simulink model "FOC"  (R2024b)
settings: Solver=FixedStepAuto  StartTime=0.0  StopTime=2.4  FixedStep=1e-5  RelTol=1e-3
values from neighbouring files (symbols this model uses):
  dam = 0.707    [data_foc_fpc_zhang.mat]
  gama = 0.9    [data_foc_fpc_zhang.mat]
  imd = [-200 -190 -180 -170 -160 -150 -140 -130 -120 -110 -100 -90 ... (41 elements, 1x41)]    [data_foc_fpc_zhang.mat]
  imq = [-200 -180 -160 -140 -120 -100 -80 -60 -40 -20 0 20 ... (21 elements, 1x21)]    [data_foc_fpc_zhang.mat]
  L_loss = 0.0001    [data_foc_fpc_zhang.mat]
  Lmidd = [0.0012418475022 0.00124844926594 0.00125505102968 0.00126370970426 0.00127249900958 0.00128126693334 0.00129343475618 0.00129881592306 0.00130559003385 0.00130625690774 0.00129596814237 0.00127902455887 ... (861 elements, 41x21)]    [data_foc_fpc_zhang.mat]
  Lmidq = [-8.03588800241e-05 -7.81376313538e-05 -7.59163826835e-05 -6.79567507785e-05 -6.10868587727e-05 -5.46820183962e-05 -4.43623922788e-05 -2.78718084301e-05 -1.24477686412e-05 4.13620151953e-06 2.37103656882e-05 4.4707150748e-05 ... (861 elements, 41x21)]    [data_foc_fpc_zhang.mat]
  Lmiqq = [0.000622544120709 0.000618884908772 0.000615225696834 0.000593520125188 0.000579858645255 0.000568946837315 0.000562248369566 0.000560456845994 0.000560437513873 0.000561933244764 0.00056023385138 0.000557379247045 ... (861 elements, 41x21)]    [data_foc_fpc_zhang.mat]
  phase_number = 3    [data_foc_fpc_zhang.mat]
  pp = 4    [data_foc_fpc_zhang.mat]
  Psid = [-0.0498528002107 -0.0378839484092 -0.0259882808465 -0.013034575748 3.54716858652e-05 0.0129865277943 0.0255980427761 0.0386444323153 0.0516254468728 0.0646548336102 0.0777195684651 0.0905974700702 ... (861 elements, 41x21)]    [data_foc_fpc_zhang.mat]
  Psiq = [-0.428836914229 -0.429385909203 -0.42997932915 -0.43118839194 -0.431809140992 -0.432336580454 -0.433057103512 -0.432963079787 -0.433296951787 -0.433632934983 -0.43343561964 -0.433301309559 ... (861 elements, 41x21)]    [data_foc_fpc_zhang.mat]
  Rs = 0.015    [data_foc_fpc_zhang.mat]
  T_ref = 162    [data_foc_fpc_zhang.mat]
  Ts = 1e-05    [data_foc_fpc_zhang.mat]
undefined symbols (not defined in the file or in its folder): DiscIntNeverNeededParam, UNC, V_dc
libraries: simulink x7, spsabctodq0Lib x2, spsdq0toabcLib x2, simulink_extras x2, mcbcontrolslib x2, mcbplantlib x1
settings Model: Creator=zhang5  LastModifiedBy=zhang5
settings DataIOCC: ReturnWorkspaceOutputs=off

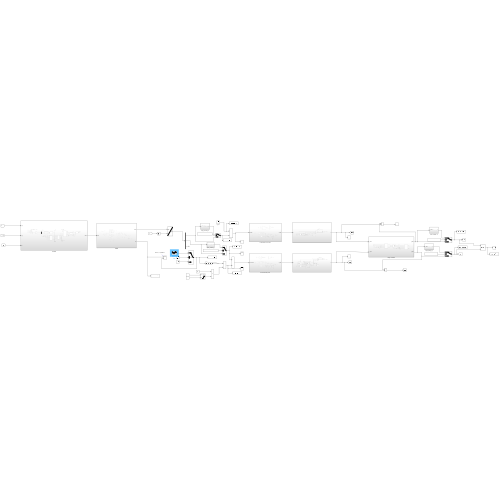
[thumbnail: Simulink's stored preview of the top-level diagram]
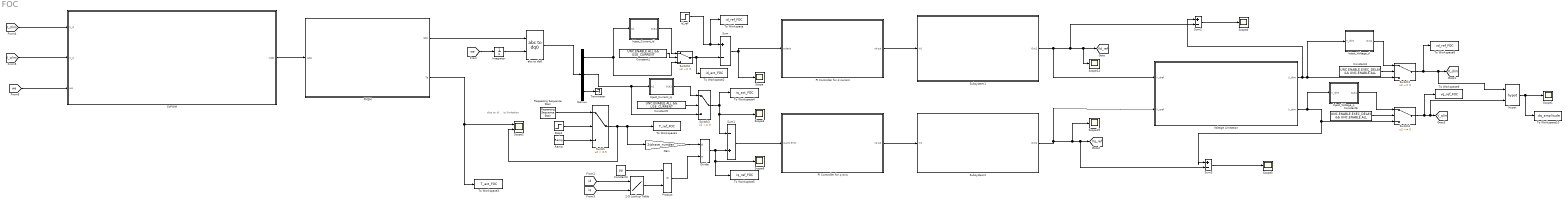
== system FOC ==
  note: due to id ， iq limitation
  2-D Lookup Table : Lookup_n-D  BreakpointsForDimension1=imd  BreakpointsForDimension2=imq  Table=Psid  InternalRulePriority=Speed  RndMeth=Simplest
      settings: InputPortMap=u0,u1
  Constant1 : Constant  Value="UNC.ENABLE.ALL   && USE_CURRENT"
  Constant3 : Constant  Value=pp
  Constant4 : Constant  Value="UNC.ENABLE.EXEC_DELAY &&  UNC.ENABLE.ALL"
  Constant5 : Constant  Value="UNC.ENABLE.ALL   && USE_CURRENT"
  Constant6 : Constant  Value=UNC.ENABLE.EXEC_DELAY && UNC.ENABLE.ALL
  Demux : Demux  Outputs=3
  Divide : Product  Inputs=*/
  Gain : Gain  Gain=2/phase_number
  Hypot : Math  Operator=hypot
  Inject_Current_id : Subsystem
  Inject_Current_iq : Subsystem
  Inject_Voltage_d : Subsystem
  Inject_Voltage_q : Subsystem
  Integrator : Integrator
  "PI Controller for d current " : Subsystem
  "PI Controller for q axis " : Subsystem
  PMSM : Subsystem
  Product : Product
  Ramp : simulink/Sources/Ramp  slope=90  start=0  InitialOutput=0
  Repeating Sequence Stair : simulink/Sources/Repeating Sequence Stair  OutValues="[T_ref  -T_ref*0.3 -T_ref*1.8 -T_ref T_ref*1.8 T_ref*0.1].'"  tsamp=0.4  OutMin=[]  OutMax=[]  OutDataTypeStr=double  OutputDataTypeScalingMode=double  OutDataType=fixdt(0,8)  ConRadixGroup=Best Precision: Vector-wise  OutScaling=2^-12
  SVPWM : Subsystem
  Scope{,1,3..6,14..15} (8 alike) : Scope
  Scope2 : Scope  NumInputPorts=2
  Step1 : Step  Time=5  SampleTime=0
  Subsystem1 : Subsystem
  Subsystem2 : Subsystem
  Sum : Sum  Inputs=+-
  Sum1 : Sum  Inputs=-+
  Sum2 : Sum  Inputs=+-
  Sum3 : Sum  Inputs=+-
  Switch : Switch  Criteria=u2 > Threshold  Threshold=0.5  SaturateOnIntegerOverflow=off  InputSameDT=off
  Switch{1..4} (4 alike) : Switch  Criteria=u2 ~= 0  SaturateOnIntegerOverflow=off  InputSameDT=off
  Terminator : Terminator
  To Workspace : ToWorkspace  VariableName=id_ref_FOC  SaveFormat=Structure With Time  SampleTime=-1
  To Workspace1 : ToWorkspace  VariableName=T_ref_FOC  SaveFormat=Structure With Time  SampleTime=-1
  To Workspace10 : ToWorkspace  VariableName=dq_amplitude  SaveFormat=Structure With Time  SampleTime=-1
  To Workspace2 : ToWorkspace  VariableName=id_act_FOC  SaveFormat=Structure With Time  SampleTime=-1
  To Workspace3 : ToWorkspace  VariableName=T_act_FOC  SaveFormat=Structure With Time  SampleTime=-1
  To Workspace4 : ToWorkspace  VariableName=iq_act_FOC  SaveFormat=Structure With Time  SampleTime=-1
  To Workspace5 : ToWorkspace  VariableName=iq_ref_FOC  SaveFormat=Structure With Time  SampleTime=-1
  To Workspace8 : ToWorkspace  VariableName=vd_ref_FOC  SaveFormat=Structure With Time  SampleTime=-1
  To Workspace9 : ToWorkspace  VariableName=vq_ref_FOC  SaveFormat=Structure With Time  SampleTime=-1
  Voltage Limitation : Subsystem
  abc to dq0 : spsabctodq0Lib/abc to dq0  Alignment=Aligned with phase A axis
  id_ref : Step  Time=4  After=0  SampleTime=0
  tag scope: V_dlim=global, V_qlim=global, Vd_ref=global, Vq_ref=global
  wires:
  [we] -> Integrator/1
  Integrator/1 -> abc to dq0/2
  abc to dq0/1 -> Demux/1
  Demux/3 -> Terminator/1
  Gain/1 -> Divide/1
  Constant3/1 -> Product/1
  [id] -> 2-D Lookup Table/1
  [iq] -> 2-D Lookup Table/2
  Product/1 -> Divide/2
  Sum/1 -> Scope/1, "PI Controller for d current "/1(e daxis)
  Sum1/1 -> "PI Controller for q axis "/1(q axis error)
  "PI Controller for d current "/1(vd out) -> Subsystem1/1(In1)
  Subsystem1/1(Out1) -> Sum2/2, Scope14/1, [Vd_ref], Voltage Limitation/1(V_dref)
  "PI Controller for q axis "/1(vq out) -> Subsystem2/1(In1)
  Voltage Limitation/1(V_dlim) -> Sum2/1, Inject_Voltage_d/1(V_dlim), Switch1/3
  Sum2/1 -> Scope4/1
  Sum3/1 -> Scope5/1
  Voltage Limitation/2(V_qlim) -> Inject_Voltage_q/1(V_dlim), Switch4/3, Sum3/1
  Subsystem2/1(Out1) -> Voltage Limitation/2(V_qref), Scope15/1, Sum3/2, [Vq_ref]
  Step1/1 -> Switch/2
  PMSM/2(Te) -> Scope2/1, To Workspace3/1
  id_ref/1 -> To Workspace/1, Sum/1
  Ramp/1 -> Switch/3
  Switch/1 -> Gain/1, To Workspace1/1, Scope2/2
  PMSM/1(iabc) -> abc to dq0/1
  Constant4/1 -> Switch1/2
  Demux/1 -> Inject_Current_id/1(In1), Switch2/3
  Demux/2 -> Switch3/3, Inject_Current_iq/1(In1)
  Constant1/1 -> Switch2/2
  Inject_Current_id/1(Out1) -> Switch2/1
  Inject_Current_iq/1(Out1) -> Switch3/1
  Constant5/1 -> Switch3/2
  Inject_Voltage_d/1(Out1) -> Switch1/1
  Inject_Voltage_q/1(Out1) -> Switch4/1
  Constant6/1 -> Switch4/2
  Switch2/1 -> To Workspace2/1, Sum/2
  Switch3/1 -> To Workspace4/1, Scope3/1, Sum1/1
  Switch1/1 -> To Workspace8/1, Hypot/1, [V_dlim]
  Switch4/1 -> To Workspace9/1, Hypot/2, [V_qlim]
  Divide/1 -> Scope6/1, To Workspace5/1, Sum1/2
  Repeating Sequence Stair/1 -> Switch/1
  [V_dlim] -> SVPWM/1(V_d)
  [V_qlim] -> SVPWM/2(V_q)
  [we] -> SVPWM/3(we)
  SVPWM/1(Vabc) -> PMSM/1(vabc)
  Hypot/1 -> To Workspace10/1, Scope1/1
  2-D Lookup Table/1 -> Product/2

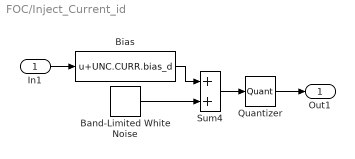
== system FOC/Inject_Current_id ==
  In1 : Inport
  Band-Limited White Noise : simulink/Sources/Band-Limited White Noise  Cov=UNC.CURR.noise_psd  Ts=1e-5  seed=[23341]
  Bias : Bias  Bias=UNC.CURR.bias_d  SaturateOnIntegerOverflow=off
  Quantizer : Quantizer  QuantizationInterval=UNC.CURR.quant
  Sum4 : Sum
  Out1 : Outport
  wires:
  Sum4/1 -> Quantizer/1
  Quantizer/1 -> Out1/1
  In1/1 -> Bias/1
  Bias/1 -> Sum4/1
  Band-Limited White Noise/1 -> Sum4/2

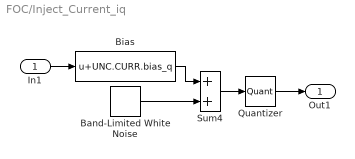
== system FOC/Inject_Current_iq ==
  In1 : Inport
  Band-Limited White Noise : simulink/Sources/Band-Limited White Noise  Cov=UNC.CURR.noise_psd  Ts=1e-5  seed=[23341]
  Bias : Bias  Bias=UNC.CURR.bias_q  SaturateOnIntegerOverflow=off
  Quantizer : Quantizer  QuantizationInterval=UNC.CURR.quant
  Sum4 : Sum
  Out1 : Outport
  wires:
  Band-Limited White Noise/1 -> Sum4/2
  Bias/1 -> Sum4/1
  In1/1 -> Bias/1
  Quantizer/1 -> Out1/1
  Sum4/1 -> Quantizer/1

== system FOC/Inject_Voltage_d ==
  V_dlim : Inport
  Transport Delay : TransportDelay  DelayTime=UNC.DELAY.ctrl
  Out1 : Outport
  wires:
  V_dlim/1 -> Transport Delay/1
  Transport Delay/1 -> Out1/1

== system FOC/Inject_Voltage_q ==
  V_dlim : Inport
  Transport Delay : TransportDelay  DelayTime=UNC.DELAY.ctrl
  Out1 : Outport
  wires:
  Transport Delay/1 -> Out1/1
  V_dlim/1 -> Transport Delay/1

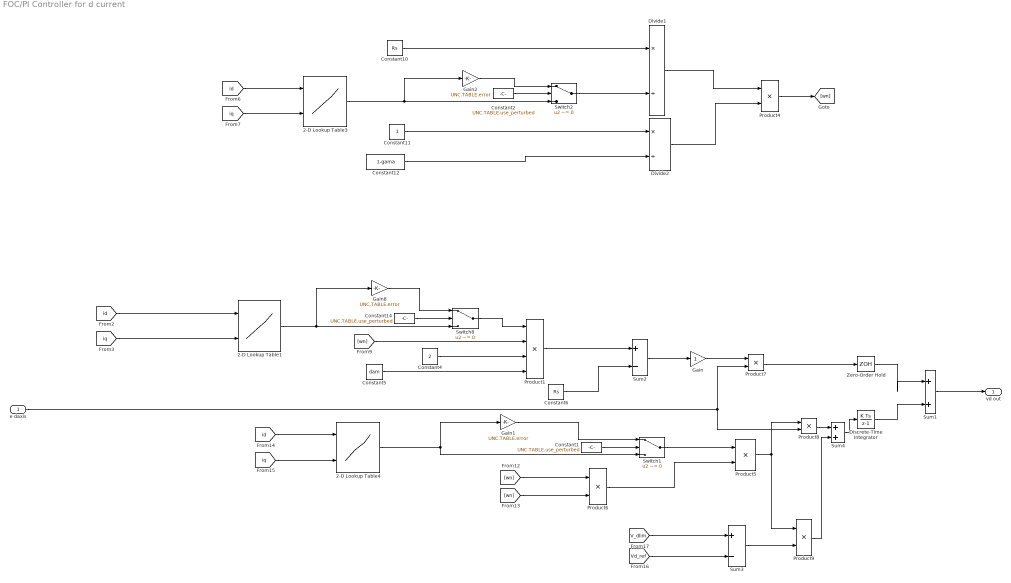
== system FOC/PI Controller for d current  ==
  e daxis : Inport
  2-D Lookup Table1 : Lookup_n-D  BreakpointsForDimension1=imd  BreakpointsForDimension2=imq  Table=Lmidd  InternalRulePriority=Speed  RndMeth=Simplest
      settings: InputPortMap=u0,u1
  2-D Lookup Table3 : Lookup_n-D  BreakpointsForDimension1=imd  BreakpointsForDimension2=imq  Table=Lmidd  InternalRulePriority=Speed  RndMeth=Simplest
      settings: InputPortMap=u0,u1
  2-D Lookup Table4 : Lookup_n-D  BreakpointsForDimension1=imd  BreakpointsForDimension2=imq  Table=Lmidd  InternalRulePriority=Speed  RndMeth=Simplest
      settings: InputPortMap=u0,u1
  Constant1 : Constant  Value=UNC.TABLE.use_perturbed
  Constant10 : Constant  Value=Rs
  Constant11 : Constant
  Constant12 : Constant  Value=1-gama
  Constant14 : Constant  Value=UNC.TABLE.use_perturbed
  Constant2 : Constant  Value=UNC.TABLE.use_perturbed
  Constant4 : Constant  Value=2
  Constant5 : Constant  Value=dam
  Constant6 : Constant  Value=Rs
  Discrete-Time Integrator : DiscreteIntegrator  SampleTime=Ts  ICPrevOutput=DiscIntNeverNeededParam  ICPrevScaledInput=DiscIntNeverNeededParam
  Divide1 : Product  Inputs=*/
  Divide2 : Product  Inputs=*/
  Gain : Gain
  Gain1 : Gain  Gain=UNC.TABLE.error
  Gain2 : Gain  Gain=UNC.TABLE.error
  Gain8 : Gain  Gain=UNC.TABLE.error
  Product1 : Product  Inputs=4
  Product{4..9} (6 alike) : Product
  Sum1 : Sum  Inputs=|++
  Sum2 : Sum  Inputs=+-
  Sum3 : Sum  Inputs=+-
  Sum4 : Sum
  Switch1 : Switch  Criteria=u2 ~= 0  SaturateOnIntegerOverflow=off  InputSameDT=off
  Switch2 : Switch  Criteria=u2 ~= 0  SaturateOnIntegerOverflow=off  InputSameDT=off
  Switch8 : Switch  Criteria=u2 ~= 0  SaturateOnIntegerOverflow=off  InputSameDT=off
  Zero-Order Hold : ZeroOrderHold  SampleTime=Ts
  vd out : Outport
  wires:
  Constant12/1 -> Divide2/2
  Divide2/1 -> Product4/2
  Constant11/1 -> Divide2/1
  Product4/1 -> [wn]
  Divide1/1 -> Product4/1
  [id] -> 2-D Lookup Table3/1
  [iq] -> 2-D Lookup Table3/2
  Constant10/1 -> Divide1/1
  Zero-Order Hold/1 -> Sum1/1
  Discrete-Time Integrator/1 -> Sum1/2
  Product1/1 -> Sum2/1
  Constant4/1 -> Product1/3
  Constant5/1 -> Product1/4
  [wn] -> Product1/2
  [id] -> 2-D Lookup Table1/1
  Constant6/1 -> Sum2/2
  [iq] -> 2-D Lookup Table1/2
  [id] -> 2-D Lookup Table4/1
  [wn] -> Product6/2
  Product6/1 -> Product5/2
  [iq] -> 2-D Lookup Table4/2
  [wn] -> Product6/1
  Sum2/1 -> Gain/1
  Product7/1 -> Zero-Order Hold/1
  Product5/1 -> Product9/1, Product8/1
  e daxis/1 -> Product7/2, Product8/2
  Sum1/1 -> vd out/1
  [Vd_ref] -> Sum3/2
  [V_dlim] -> Sum3/1
  Sum3/1 -> Product9/2
  Product8/1 -> Sum4/1
  Product9/1 -> Sum4/2
  Sum4/1 -> Discrete-Time Integrator/1
  Gain/1 -> Product7/1
  Constant14/1 -> Switch8/2
  Gain8/1 -> Switch8/1
  2-D Lookup Table1/1 -> Gain8/1, Switch8/3
  Switch8/1 -> Product1/1
  Switch1/1 -> Product5/1
  2-D Lookup Table4/1 -> Switch1/3, Gain1/1
  Gain1/1 -> Switch1/1
  Constant1/1 -> Switch1/2
  Switch2/1 -> Divide1/2
  2-D Lookup Table3/1 -> Switch2/3, Gain2/1
  Gain2/1 -> Switch2/1
  Constant2/1 -> Switch2/2

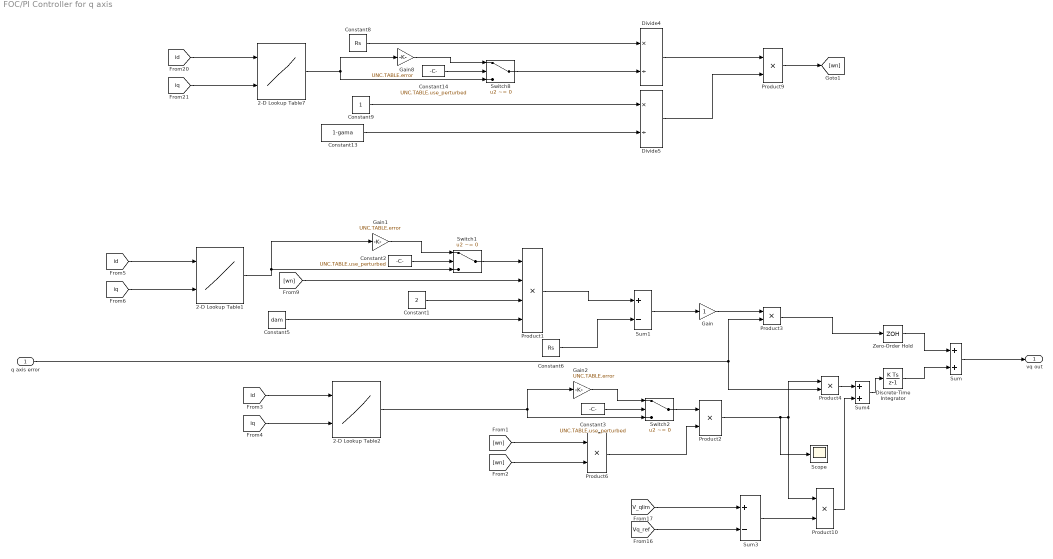
== system FOC/PI Controller for q axis  ==
  q axis error : Inport
  2-D Lookup Table1 : Lookup_n-D  BreakpointsForDimension1=imd  BreakpointsForDimension2=imq  Table=Lmiqq  InternalRulePriority=Speed  RndMeth=Simplest
      settings: InputPortMap=u0,u1
  2-D Lookup Table2 : Lookup_n-D  BreakpointsForDimension1=imd  BreakpointsForDimension2=imq  Table=Lmiqq  InternalRulePriority=Speed  RndMeth=Simplest
      settings: InputPortMap=u0,u1
  2-D Lookup Table7 : Lookup_n-D  BreakpointsForDimension1=imd  BreakpointsForDimension2=imq  Table=Lmiqq  InternalRulePriority=Speed  RndMeth=Simplest
      settings: InputPortMap=u0,u1
  Constant1 : Constant  Value=2
  Constant13 : Constant  Value=1-gama
  Constant14 : Constant  Value=UNC.TABLE.use_perturbed
  Constant2 : Constant  Value=UNC.TABLE.use_perturbed
  Constant3 : Constant  Value=UNC.TABLE.use_perturbed
  Constant5 : Constant  Value=dam
  Constant6 : Constant  Value=Rs
  Constant8 : Constant  Value=Rs
  Constant9 : Constant
  Discrete-Time Integrator : DiscreteIntegrator  SampleTime=Ts  ICPrevOutput=DiscIntNeverNeededParam  ICPrevScaledInput=DiscIntNeverNeededParam
  Divide4 : Product  Inputs=*/
  Divide5 : Product  Inputs=*/
  Gain : Gain
  Gain1 : Gain  Gain=UNC.TABLE.error
  Gain2 : Gain  Gain=UNC.TABLE.error
  Gain8 : Gain  Gain=UNC.TABLE.error
  Product1 : Product  Inputs=4
  Product{2..4,6,9..10} (6 alike) : Product
  Scope : Scope
  Sum : Sum
  Sum1 : Sum  Inputs=+-
  Sum3 : Sum  Inputs=+-
  Sum4 : Sum
  Switch1 : Switch  Criteria=u2 ~= 0  SaturateOnIntegerOverflow=off  InputSameDT=off
  Switch2 : Switch  Criteria=u2 ~= 0  SaturateOnIntegerOverflow=off  InputSameDT=off
  Switch8 : Switch  Criteria=u2 ~= 0  SaturateOnIntegerOverflow=off  InputSameDT=off
  Zero-Order Hold : ZeroOrderHold  SampleTime=Ts
  vq out : Outport
  wires:
  Constant13/1 -> Divide5/2
  Divide4/1 -> Product9/1
  Product9/1 -> [wn]
  Constant9/1 -> Divide5/1
  [id] -> 2-D Lookup Table7/1
  Constant8/1 -> Divide4/1
  Divide5/1 -> Product9/2
  [iq] -> 2-D Lookup Table7/2
  Sum4/1 -> Discrete-Time Integrator/1
  q axis error/1 -> Product4/2, Product3/2
  Zero-Order Hold/1 -> Sum/1
  Constant6/1 -> Sum1/2
  Discrete-Time Integrator/1 -> Sum/2
  Constant5/1 -> Product1/4
  Constant1/1 -> Product1/3
  [wn] -> Product1/2
  Product1/1 -> Sum1/1
  Sum3/1 -> Product10/2
  Product2/1 -> Scope/1, Product10/1, Product4/1
  [V_qlim] -> Sum3/1
  Product10/1 -> Sum4/2
  Sum1/1 -> Gain/1
  [Vq_ref] -> Sum3/2
  [wn] -> Product6/2
  [wn] -> Product6/1
  Product6/1 -> Product2/2
  Product4/1 -> Sum4/1
  Product3/1 -> Zero-Order Hold/1
  [iq] -> 2-D Lookup Table1/2
  [id] -> 2-D Lookup Table1/1
  [iq] -> 2-D Lookup Table2/2
  [id] -> 2-D Lookup Table2/1
  Sum/1 -> vq out/1
  Gain/1 -> Product3/1
  Constant14/1 -> Switch8/2
  Gain8/1 -> Switch8/1
  2-D Lookup Table7/1 -> Gain8/1, Switch8/3
  Switch8/1 -> Divide4/2
  2-D Lookup Table1/1 -> Gain1/1, Switch1/3
  Gain1/1 -> Switch1/1
  Constant2/1 -> Switch1/2
  Constant3/1 -> Switch2/2
  Gain2/1 -> Switch2/1
  2-D Lookup Table2/1 -> Switch2/3, Gain2/1
  Switch2/1 -> Product2/1
  Switch1/1 -> Product1/1

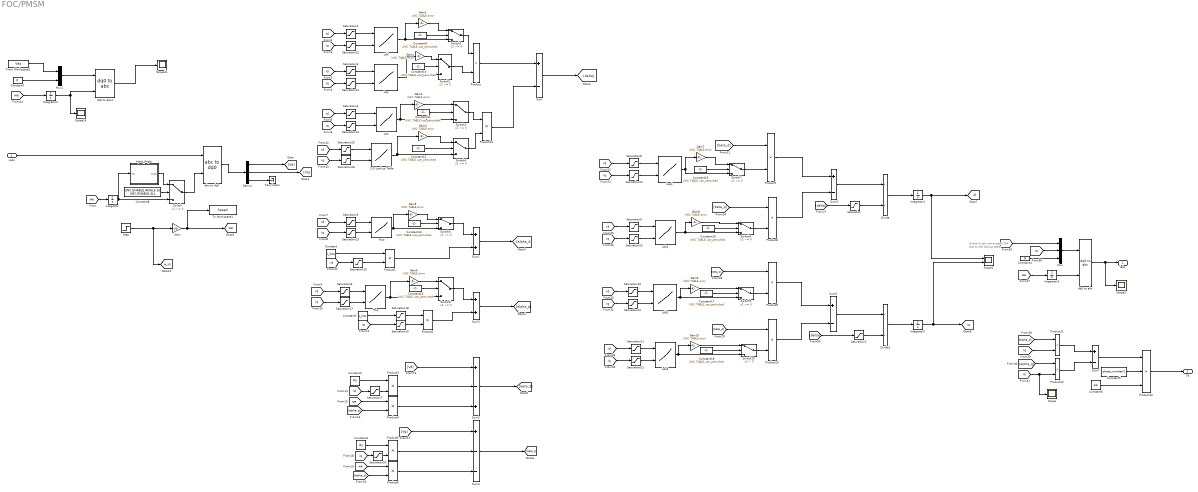
== system FOC/PMSM ==
  note: id and iq can not exceed 200
      | due to the lookup table
  vabc : Inport
  2-D Lookup Table : Lookup_n-D  BreakpointsForDimension1=imd  BreakpointsForDimension2=imq  Table=Lmidq  ExtrapMethod=Clip  UseLastTableValue=on  InternalRulePriority=Speed  RndMeth=Simplest
      settings: InputPortMap=u0,u1
  Constant : Constant  Value=L_loss
  Constant1 : Constant  Value=L_loss
  Constant{9..18} (10 alike) : Constant  Value=UNC.TABLE.use_perturbed
  Constant2 : Constant  Value=Rs
  Constant3 : Constant  Value=Rs
  Constant4 : Constant  Value=0
  Constant5 : Constant  Value=phase_number/2
  Constant6 : Constant  Value=pp
  Constant7 : Constant  Value=0
  Constant8 : Constant  Value=UNC.ENABLE.ANGLE && UNC.ENABLE.ALL
  Demux : Demux  Outputs=3
  Divide : Product  Inputs=*/
  Divide1 : Product  Inputs=*/
  From Workspace2 : FromWorkspace  VariableName=Vdq  SampleTime=1e-5  Interpolate=off  OutputAfterFinalValue=Holding final value
  Gain : Gain  Gain=pp
  Gain{1..10} (10 alike) : Gain  Gain=UNC.TABLE.error
  Inject_Angle : Subsystem
  Integrator : Integrator  UpperSaturationLimit=pi  LowerSaturationLimit=-pi
  Integrator1 : Integrator
  Integrator2 : Integrator
  Integrator3 : Integrator  UpperSaturationLimit=pi  LowerSaturationLimit=-pi
  Integrator4 : Integrator  UpperSaturationLimit=pi  LowerSaturationLimit=-pi
  Ldd : Lookup_n-D  BreakpointsForDimension1=imd  BreakpointsForDimension2=imq  Table=Lmidd  ExtrapMethod=Clip  UseLastTableValue=on  InternalRulePriority=Speed  RndMeth=Simplest
      settings: InputPortMap=u0,u1
  Ldd1 : Lookup_n-D  BreakpointsForDimension1=imd  BreakpointsForDimension2=imq  Table=Lmidd  ExtrapMethod=Clip  UseLastTableValue=on  InternalRulePriority=Speed  RndMeth=Simplest
      settings: InputPortMap=u0,u1
  Ldq : Lookup_n-D  BreakpointsForDimension1=imd  BreakpointsForDimension2=imq  Table=Lmidq  ExtrapMethod=Clip  UseLastTableValue=on  InternalRulePriority=Speed  RndMeth=Simplest
      settings: InputPortMap=u0,u1
  Ldq1 : Lookup_n-D  BreakpointsForDimension1=imd  BreakpointsForDimension2=imq  Table=Lmidq  ExtrapMethod=Clip  UseLastTableValue=on  InternalRulePriority=Speed  RndMeth=Simplest
      settings: InputPortMap=u0,u1
  Ldq2 : Lookup_n-D  BreakpointsForDimension1=imd  BreakpointsForDimension2=imq  Table=Lmidq  ExtrapMethod=Clip  UseLastTableValue=on  InternalRulePriority=Speed  RndMeth=Simplest
      settings: InputPortMap=u0,u1
  Lqq : Lookup_n-D  BreakpointsForDimension1=imd  BreakpointsForDimension2=imq  Table=Lmiqq  ExtrapMethod=Clip  UseLastTableValue=on  InternalRulePriority=Speed  RndMeth=Simplest
      settings: InputPortMap=u0,u1
  Lqq1 : Lookup_n-D  BreakpointsForDimension1=imd  BreakpointsForDimension2=imq  Table=Lmiqq  ExtrapMethod=Clip  UseLastTableValue=on  InternalRulePriority=Speed  RndMeth=Simplest
      settings: InputPortMap=u0,u1
  Mux : Mux  Inputs=3
  Mux1 : Mux  Inputs=2
  Product{,1..12,14} (14 alike) : Product
  Product13 : Product  Inputs=3
  Psid : Lookup_n-D  BreakpointsForDimension1=imd  BreakpointsForDimension2=imq  Table=Psid  ExtrapMethod=Clip  UseLastTableValue=on  InternalRulePriority=Speed  RndMeth=Simplest
      settings: InputPortMap=u0,u1
  Psiq : Lookup_n-D  BreakpointsForDimension1=imd  BreakpointsForDimension2=imq  Table=Psiq  ExtrapMethod=Clip  UseLastTableValue=on  InternalRulePriority=Speed  RndMeth=Simplest
      settings: InputPortMap=u0,u1
  Saturation : Saturate  UpperLimit=10000000000000000000000  LowerLimit=1e-6
  Saturation1 : Saturate  UpperLimit=10000000000000000000000  LowerLimit=1e-6
  Saturation{2..11,13..26} (24 alike) : Saturate  UpperLimit=200  LowerLimit=-200
  Saturation12 : Saturate
  Scope{,2,11,14} (4 alike) : Scope
  Scope1 : Scope  NumInputPorts=2
  Step : Step  Time=5  Before=10.4720  After=10.4720*1.2  SampleTime=0
  Sum{,5..7} (4 alike) : Sum  Inputs=+-
  Sum1 : Sum
  Sum2 : Sum
  Sum3 : Sum  Inputs=+-+
  Sum4 : Sum  Inputs=+--
  Switch{,1..9} (10 alike) : Switch  Criteria=u2 ~= 0  SaturateOnIntegerOverflow=off  InputSameDT=off
  Switch10 : Switch  Criteria=u2 > Threshold  SaturateOnIntegerOverflow=off  InputSameDT=off
  Terminator : Terminator
  To Workspace1 : ToWorkspace  VariableName=Speed  SaveFormat=Structure With Time  SampleTime=-1
  abc to dq0 : spsabctodq0Lib/abc to dq0  Alignment=Aligned with phase A axis
  dq0 to abc : spsdq0toabcLib/dq0 to abc  Alignment=Aligned with phase A axis
  dq0 to abc1 : spsdq0toabcLib/dq0 to abc  Alignment=Aligned with phase A axis
  iabc : Outport
  Te : Outport  Port=2
  tag scope: id=global, iq=global, w_m=global, we=global
  wires:
  [iq] -> Saturation17/1
  [iq] -> Saturation12/1
  [iq] -> Saturation21/1
  Constant2/1 -> Product3/1
  Product4/1 -> Sum3/3
  [iq] -> Saturation19/1
  [iq] -> Saturation15/1
  [id] -> Saturation16/1
  Constant3/1 -> Product5/1
  [id] -> Saturation2/1
  [beta_d] -> Product10/1
  [we] -> Integrator/1
  [id] -> Saturation10/1
  Demux/3 -> Terminator/1
  dq0 to abc/1 -> Scope2/1, iabc/1
  Constant4/1 -> Mux/3
  [id] -> Saturation6/1
  [Vq] -> Sum4/1
  Divide1/1 -> Integrator2/1
  [alpha_d] -> Product6/2
  [iq] -> Saturation14/1
  Mux/1 -> dq0 to abc/1
  [id] -> Saturation9/1
  Product6/1 -> Sum4/3
  [iq] -> Saturation13/1
  [id] -> Saturation3/1
  [iq] -> Saturation24/1
  Product7/1 -> Sum5/1
  Sum2/1 -> [alpha_q]
  Product14/1 -> Sum/2
  [id] -> Saturation4/1
  [iq] -> Saturation20/1
  [we] -> Integrator3/1
  [delta] -> Saturation/1
  [id] -> Saturation7/1
  Sum5/1 -> Divide/1
  Product8/1 -> Sum5/2
  Product3/1 -> Sum3/2
  Gain/1 -> To Workspace1/1, [we]
  [beta_q] -> Product8/1
  Integrator3/1 -> dq0 to abc/2
  [beta_d] -> Product7/1
  [id] -> Saturation8/1
  [iq] -> Mux/2
  Divide/1 -> Integrator1/1
  Product9/1 -> Sum6/1
  Product5/1 -> Sum4/2
  Constant1/1 -> Saturation18/1
  Product10/1 -> Sum6/2
  [id] -> Mux/1
  [we] -> Product4/1
  [iq] -> Saturation23/1
  Product/1 -> Sum/1
  Sum6/1 -> Divide1/1
  [we] -> Product6/1
  Sum3/1 -> [beta_d]
  [alpha_q] -> Product4/2
  Sum4/1 -> [beta_q]
  Sum1/1 -> [alpha_d]
  [id] -> Saturation11/1
  [id] -> Saturation5/1
  [Vd] -> Sum3/1
  [delta] -> Saturation1/1
  Integrator1/1 -> Scope1/1, [id]
  Constant/1 -> Product1/1
  Sum/1 -> [delta]
  [iq] -> Saturation22/1
  [beta_q] -> Product9/1
  [alpha_d] -> Product11/1
  [iq] -> Product11/2
  Product11/1 -> Sum7/1
  [alpha_q] -> Product12/1
  [id] -> Scope/1, Product12/2
  Product12/1 -> Sum7/2
  Sum7/1 -> Product13/1
  Constant5/1 -> Product13/2
  Constant6/1 -> Product13/3
  Product13/1 -> Te/1
  Saturation/1 -> Divide/2
  Saturation1/1 -> Divide1/2
  Saturation2/1 -> Ldd/1
  Saturation3/1 -> Lqq/1
  Saturation4/1 -> Ldq/1
  Saturation5/1 -> Psid/1
  Saturation6/1 -> Psiq/1
  Saturation7/1 -> Product3/2
  Saturation8/1 -> Lqq1/1
  Saturation9/1 -> Ldq1/1
  Saturation10/1 -> Ldd1/1
  Saturation11/1 -> Ldq2/1
  Saturation12/1 -> Ldd/2
  Saturation13/1 -> Lqq/2
  Saturation14/1 -> Ldq/2
  Saturation15/1 -> Psid/2
  Saturation16/1 -> Product1/2
  Saturation17/1 -> Psiq/2
  Saturation18/1 -> Product2/1
  Saturation19/1 -> Product2/2
  Saturation20/1 -> Product5/2
  Saturation21/1 -> Ldq2/2
  Saturation22/1 -> Ldd1/2
  Saturation23/1 -> Ldq1/2
  Saturation24/1 -> Lqq1/2
  [id] -> Saturation25/1
  [iq] -> Saturation26/1
  Saturation25/1 -> 2-D Lookup Table/1
  Saturation26/1 -> 2-D Lookup Table/2
  Product2/1 -> Sum2/2
  Demux/1 -> [Vd]
  Demux/2 -> [Vq]
  abc to dq0/1 -> Demux/1
  Product1/1 -> Sum1/2
  Mux1/1 -> dq0 to abc1/1
  Integrator4/1 -> Scope14/1, dq0 to abc1/2
  Constant7/1 -> Mux1/2
  From Workspace2/1 -> Mux1/1
  dq0 to abc1/1 -> Scope11/1
  [we] -> Integrator4/1
  vabc/1 -> abc to dq0/1
  Step/1 -> [w_m], Gain/1
  Integrator/1 -> Inject_Angle/1(In1), Switch/3
  Lqq/1 -> Gain2/1, Switch2/3
  Ldq/1 -> Gain3/1, Switch3/3
  2-D Lookup Table/1 -> Gain4/1, Switch4/3
  Psiq/1 -> Gain6/1, Switch6/3
  Lqq1/1 -> Gain7/1, Switch7/3
  Ldq1/1 -> Gain8/1, Switch8/3
  Ldd1/1 -> Gain9/1, Switch9/3
  Ldq2/1 -> Gain10/1, Switch10/3
  Inject_Angle/1(Out1) -> Switch/1
  Constant8/1 -> Switch/2
  Ldd/1 -> Gain1/1, Switch1/3
  Constant9/1 -> Switch1/2
  Gain1/1 -> Switch1/1
  Gain2/1 -> Switch2/1
  Switch2/1 -> Product/2
  Switch1/1 -> Product/1
  Constant10/1 -> Switch2/2
  Gain3/1 -> Switch3/1
  Switch3/1 -> Product14/1
  Constant11/1 -> Switch3/2
  Switch4/1 -> Product14/2
  Gain4/1 -> Switch4/1
  Constant12/1 -> Switch4/2
  Gain5/1 -> Switch5/1
  Psid/1 -> Gain5/1, Switch5/3
  Constant13/1 -> Switch5/2
  Gain6/1 -> Switch6/1
  Constant14/1 -> Switch6/2
  Switch6/1 -> Sum2/1
  Switch5/1 -> Sum1/1
  Gain7/1 -> Switch7/1
  Constant15/1 -> Switch7/2
  Gain8/1 -> Switch8/1
  Constant16/1 -> Switch8/2
  Gain9/1 -> Switch9/1
  Constant17/1 -> Switch9/2
  Switch9/1 -> Product9/2
  Switch8/1 -> Product8/2
  Switch10/1 -> Product10/2
  Gain10/1 -> Switch10/1
  Constant18/1 -> Switch10/2
  Switch7/1 -> Product7/2
  Switch/1 -> abc to dq0/2
  Integrator2/1 -> [iq], Scope1/2

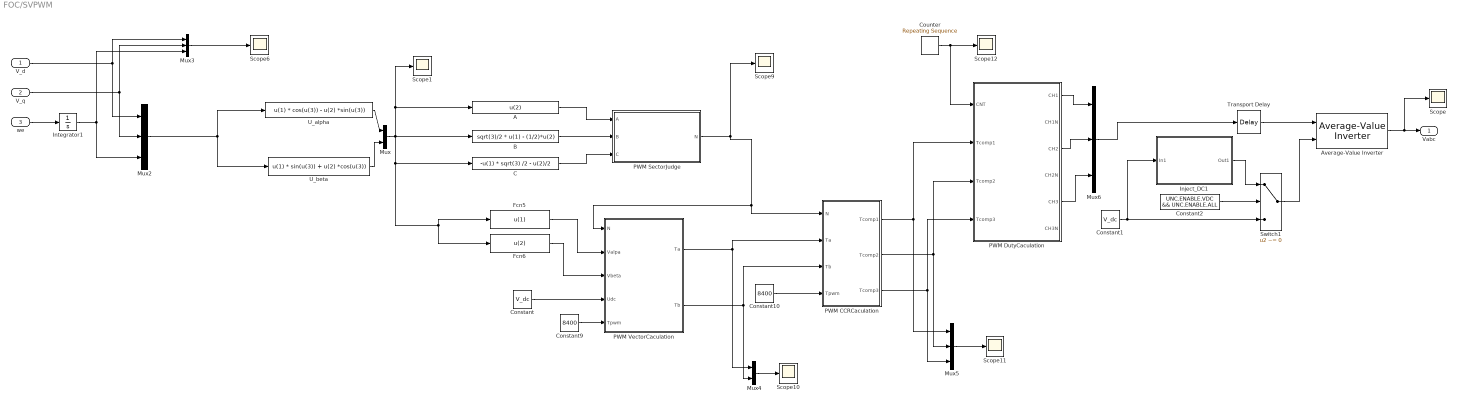
== system FOC/SVPWM ==
  V_d : Inport
  V_q : Inport  Port=2
  we : Inport  Port=3
  A : Fcn  Expr=u(2)
  Average-Value Inverter : mcbplantlib/Average-Value Inverter
      settings: LibrarySourceBlock=mcblib/Electrical Systems/Inverters/Average-Value Inverter
  B : Fcn  Expr=sqrt(3)/2 * u(1) - (1/2)*u(2)
  C : Fcn  Expr=-u(1) * sqrt(3) /2 - u(2)/2
  Constant : Constant  Value=V_dc
  Constant1 : Constant  Value=V_dc
  Constant10 : Constant  Value=8400
  Constant2 : Constant  Value=UNC.ENABLE.VDC && UNC.ENABLE.ALL
  Constant9 : Constant  Value=8400
  Counter : simulink/Sources/Repeating Sequence  rep_seq_t=[0 0.00025 0.0005]  rep_seq_y=[0 4200 0]
  Fcn5 : Fcn  Expr=u(1)
  Fcn6 : Fcn  Expr=u(2)
  Inject_DC1 : Subsystem
  Integrator1 : Integrator
  Mux : Mux  Inputs=2
  Mux{2..3,5..6} (4 alike) : Mux  Inputs=3
  Mux4 : Mux  Inputs=2
  PWM CCRCaculation : MATLAB Function  TreatAsAtomicUnit=on
  PWM DutyCaculation : MATLAB Function  TreatAsAtomicUnit=on
  PWM SectorJudge : MATLAB Function  TreatAsAtomicUnit=on
  PWM VectorCaculation : MATLAB Function  TreatAsAtomicUnit=on
  Scope{,1,6,9..12} (7 alike) : Scope
  Switch1 : Switch  Criteria=u2 ~= 0  SaturateOnIntegerOverflow=off  InputSameDT=off
  Transport Delay : TransportDelay  DelayTime=UNC.DELAY.ctrl
  U_alpha : Fcn  Expr=u(1) * cos(u(3)) - u(2) *sin(u(3))
  U_beta : Fcn  Expr=u(1) * sin(u(3)) + u(2) *cos(u(3))
  Vabc : Outport
  wires:
  Constant/1 -> PWM VectorCaculation/4(Udc)
  PWM VectorCaculation/1(Ta) -> Mux4/1, PWM CCRCaculation/2(Ta)
  U_beta/1 -> Mux/2
  Mux6/1 -> Transport Delay/1
  PWM DutyCaculation/5(CH3) -> Mux6/3
  V_d/1 -> Mux2/1, Mux3/1
  A/1 -> PWM SectorJudge/1(A)
  Integrator1/1 -> Mux2/3, Mux3/3
  Mux/1 -> Fcn6/1, Fcn5/1, C/1, Scope1/1, A/1, B/1
  PWM SectorJudge/1(N) -> PWM VectorCaculation/1(N), PWM CCRCaculation/1(N), Scope9/1
  Fcn5/1 -> PWM VectorCaculation/2(Valpa)
  PWM CCRCaculation/2(Tcomp2) -> PWM DutyCaculation/3(Tcomp2), Mux5/2
  C/1 -> PWM SectorJudge/3(C)
  PWM VectorCaculation/2(Tb) -> PWM CCRCaculation/3(Tb), Mux4/2
  PWM DutyCaculation/3(CH2) -> Mux6/2
  B/1 -> PWM SectorJudge/2(B)
  Counter/1 -> PWM DutyCaculation/1(CNT), Scope12/1
  Mux3/1 -> Scope6/1
  PWM CCRCaculation/3(Tcomp3) -> PWM DutyCaculation/4(Tcomp3), Mux5/3
  Fcn6/1 -> PWM VectorCaculation/3(Vbeta)
  Mux4/1 -> Scope10/1
  Constant9/1 -> PWM VectorCaculation/5(Tpwm)
  Mux5/1 -> Scope11/1
  PWM DutyCaculation/1(CH1) -> Mux6/1
  V_q/1 -> Mux2/2, Mux3/2
  Mux2/1 -> U_beta/1, U_alpha/1
  PWM CCRCaculation/1(Tcomp1) -> PWM DutyCaculation/2(Tcomp1), Mux5/1
  U_alpha/1 -> Mux/1
  Constant10/1 -> PWM CCRCaculation/4(Tpwm)
  we/1 -> Integrator1/1
  Average-Value Inverter/1 -> Scope/1, Vabc/1
  Inject_DC1/1(Out1) -> Switch1/1
  Switch1/1 -> Average-Value Inverter/2
  Constant2/1 -> Switch1/2
  Constant1/1 -> Inject_DC1/1(In1), Switch1/3
  Transport Delay/1 -> Average-Value Inverter/1

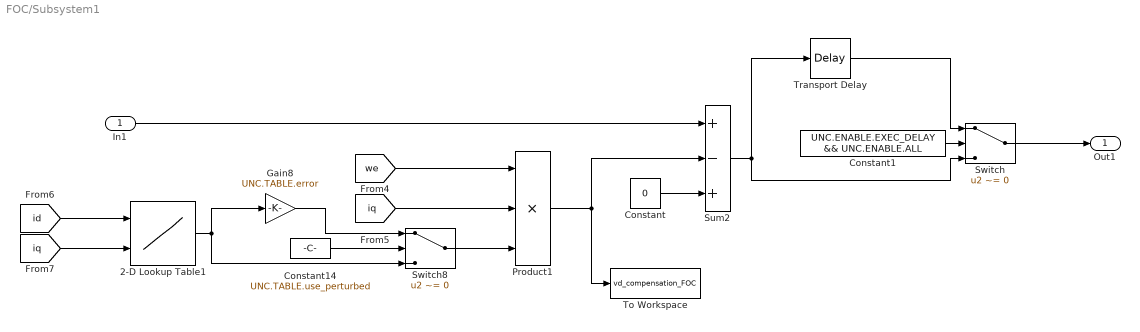
== system FOC/Subsystem1 ==
  In1 : Inport
  2-D Lookup Table1 : Lookup_n-D  BreakpointsForDimension1=imd  BreakpointsForDimension2=imq  Table=Lmiqq  InternalRulePriority=Speed  RndMeth=Simplest
      settings: InputPortMap=u0,u1
  Constant : Constant  Value=0
  Constant1 : Constant  Value=UNC.ENABLE.EXEC_DELAY && UNC.ENABLE.ALL
  Constant14 : Constant  Value=UNC.TABLE.use_perturbed
  Gain8 : Gain  Gain=UNC.TABLE.error
  Product1 : Product  Inputs=3
  Sum2 : Sum  Inputs=+-+
  Switch : Switch  Criteria=u2 ~= 0  SaturateOnIntegerOverflow=off  InputSameDT=off
  Switch8 : Switch  Criteria=u2 ~= 0  SaturateOnIntegerOverflow=off  InputSameDT=off
  To Workspace : ToWorkspace  VariableName=vd_compensation_FOC  SaveFormat=Structure With Time  SampleTime=-1
  Transport Delay : TransportDelay  DelayTime=UNC.DELAY.ff
  Out1 : Outport
  wires:
  Product1/1 -> To Workspace/1, Sum2/2
  [iq] -> 2-D Lookup Table1/2
  [iq] -> Product1/2
  [id] -> 2-D Lookup Table1/1
  [we] -> Product1/1
  In1/1 -> Sum2/1
  Constant/1 -> Sum2/3
  Constant1/1 -> Switch/2
  Sum2/1 -> Transport Delay/1, Switch/3
  Switch/1 -> Out1/1
  Transport Delay/1 -> Switch/1
  Switch8/1 -> Product1/3
  Constant14/1 -> Switch8/2
  Gain8/1 -> Switch8/1
  2-D Lookup Table1/1 -> Switch8/3, Gain8/1

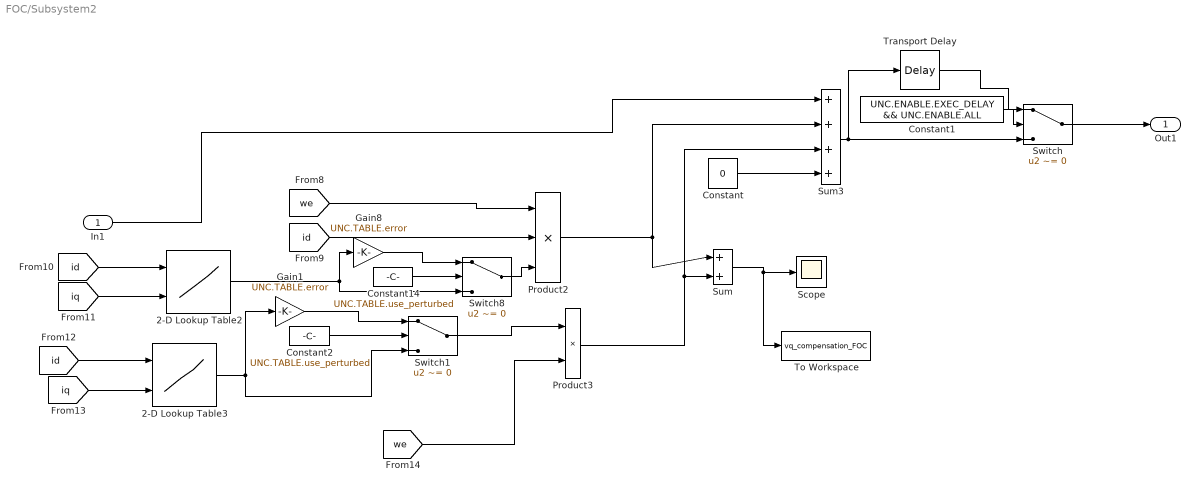
== system FOC/Subsystem2 ==
  In1 : Inport
  2-D Lookup Table2 : Lookup_n-D  BreakpointsForDimension1=imd  BreakpointsForDimension2=imq  Table=Lmidd  InternalRulePriority=Speed  RndMeth=Simplest
      settings: InputPortMap=u0,u1
  2-D Lookup Table3 : Lookup_n-D  BreakpointsForDimension1=imd  BreakpointsForDimension2=imq  Table=Psid  InternalRulePriority=Speed  RndMeth=Simplest
      settings: InputPortMap=u0,u1
  Constant : Constant  Value=0
  Constant1 : Constant  Value=UNC.ENABLE.EXEC_DELAY && UNC.ENABLE.ALL
  Constant14 : Constant  Value=UNC.TABLE.use_perturbed
  Constant2 : Constant  Value=UNC.TABLE.use_perturbed
  Gain1 : Gain  Gain=UNC.TABLE.error
  Gain8 : Gain  Gain=UNC.TABLE.error
  Product2 : Product  Inputs=3
  Product3 : Product
  Scope : Scope
  Sum : Sum  Inputs=|++
  Sum3 : Sum  Inputs=++++
  Switch : Switch  Criteria=u2 ~= 0  SaturateOnIntegerOverflow=off  InputSameDT=off
  Switch1 : Switch  Criteria=u2 ~= 0  SaturateOnIntegerOverflow=off  InputSameDT=off
  Switch8 : Switch  Criteria=u2 ~= 0  SaturateOnIntegerOverflow=off  InputSameDT=off
  To Workspace : ToWorkspace  VariableName=vq_compensation_FOC  SaveFormat=Structure With Time  SampleTime=-1
  Transport Delay : TransportDelay  DelayTime=UNC.DELAY.ff
  Out1 : Outport
  wires:
  [iq] -> 2-D Lookup Table2/2
  [iq] -> 2-D Lookup Table3/2
  Product2/1 -> Sum/1, Sum3/2
  [we] -> Product3/2
  [id] -> 2-D Lookup Table3/1
  [id] -> 2-D Lookup Table2/1
  [we] -> Product2/1
  [id] -> Product2/2
  Product3/1 -> Sum/2, Sum3/3
  In1/1 -> Sum3/1
  Constant/1 -> Sum3/4
  Sum3/1 -> Transport Delay/1, Switch/3
  Switch/1 -> Out1/1
  Transport Delay/1 -> Switch/1
  Constant1/1 -> Switch/2
  Constant14/1 -> Switch8/2
  Gain8/1 -> Switch8/1
  2-D Lookup Table2/1 -> Switch8/3, Gain8/1
  Switch8/1 -> Product2/3
  2-D Lookup Table3/1 -> Gain1/1, Switch1/3
  Gain1/1 -> Switch1/1
  Constant2/1 -> Switch1/2
  Switch1/1 -> Product3/1
  Sum/1 -> To Workspace/1, Scope/1

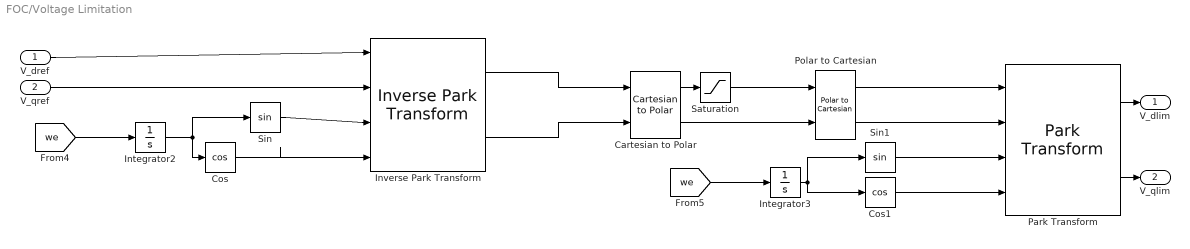
== system FOC/Voltage Limitation ==
  V_dref : Inport
  V_qref : Inport  Port=2
  Cartesian to Polar : simulink_extras/Transformations/Cartesian to Polar
  Cos : Trigonometry  Operator=cos
  Cos1 : Trigonometry  Operator=cos
  Integrator2 : Integrator
  Integrator3 : Integrator
  Inverse Park Transform : mcbcontrolslib/Inverse Park Transform  PhaseInput=Two inputs  AxisAlignment=D-axis  ThetaInput=Sine and Cosine electrical position  AngleInput=Per-unit  N_points=1024
      settings: LibrarySourceBlock=mcblib/Controls/Math Transforms/Inverse Park Transform
  Park Transform : mcbcontrolslib/Park Transform  PhaseInput=Two inputs  AxisAlignment=D-axis  ThetaInput=Sine and Cosine electrical position  AngleInput=Per-unit  N_points=1024
      settings: LibrarySourceBlock=mcblib/Controls/Math Transforms/Park Transform
  Polar to Cartesian : simulink_extras/Transformations/Polar to Cartesian
  Saturation : Saturate  UpperLimit=V_dc  LowerLimit=0
  Sin : Trigonometry
  Sin1 : Trigonometry
  V_dlim : Outport
  V_qlim : Outport  Port=2
  wires:
  Integrator2/1 -> Cos/1, Sin/1
  Integrator3/1 -> Sin1/1, Cos1/1
  [we] -> Integrator2/1
  V_dref/1 -> Inverse Park Transform/1
  Sin1/1 -> Park Transform/3
  V_qref/1 -> Inverse Park Transform/2
  Cartesian to Polar/1 -> Saturation/1
  [we] -> Integrator3/1
  Cos1/1 -> Park Transform/4
  Park Transform/2 -> V_qlim/1
  Inverse Park Transform/2 -> Cartesian to Polar/2
  Sin/1 -> Inverse Park Transform/3
  Inverse Park Transform/1 -> Cartesian to Polar/1
  Saturation/1 -> Polar to Cartesian/1
  Polar to Cartesian/1 -> Park Transform/1
  Polar to Cartesian/2 -> Park Transform/2
  Cartesian to Polar/2 -> Polar to Cartesian/2
  Cos/1 -> Inverse Park Transform/4
  Park Transform/1 -> V_dlim/1

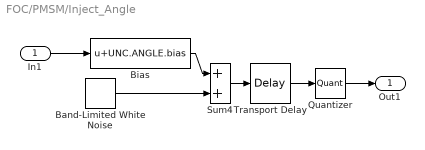
== system FOC/PMSM/Inject_Angle ==
  In1 : Inport
  Band-Limited White Noise : simulink/Sources/Band-Limited White Noise  Cov=UNC.ANGLE.noise  Ts=1e-5  seed=[23341]
  Bias : Bias  Bias=UNC.ANGLE.bias  SaturateOnIntegerOverflow=off
  Quantizer : Quantizer  QuantizationInterval=UNC.ANGLE.quant
  Sum4 : Sum
  Transport Delay : TransportDelay  DelayTime=UNC.ANGLE.delay
  Out1 : Outport
  wires:
  Band-Limited White Noise/1 -> Sum4/2
  Bias/1 -> Sum4/1
  In1/1 -> Bias/1
  Quantizer/1 -> Out1/1
  Sum4/1 -> Transport Delay/1
  Transport Delay/1 -> Quantizer/1

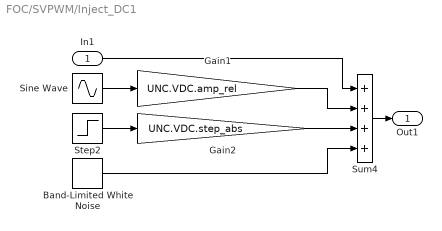
== system FOC/SVPWM/Inject_DC1 ==
  In1 : Inport
  Band-Limited White Noise : simulink/Sources/Band-Limited White Noise  Cov=UNC.VDC.noise  Ts=1e-5  seed=[23341]
  Gain1 : Gain  Gain=UNC.VDC.amp_rel
  Gain2 : Gain  Gain=UNC.VDC.step_abs
  Sine Wave : Sin  Frequency=2*pi*120  SampleTime=0
  Step2 : Step  Time=0.05  SampleTime=0
  Sum4 : Sum  Inputs=++++
  Out1 : Outport
  wires:
  In1/1 -> Sum4/1
  Gain2/1 -> Sum4/3
  Sine Wave/1 -> Gain1/1
  Step2/1 -> Gain2/1
  Gain1/1 -> Sum4/2
  Band-Limited White Noise/1 -> Sum4/4
  Sum4/1 -> Out1/1

== matlab function FOC/SVPWM/PWM DutyCaculation ==
  data: CNT input; CH1 output; Tcomp1 input; Tcomp2 input; Tcomp3 input; CH1N output; CH2 output; CH2N output; CH3 output; CH3N output
function [CH1, CH1N, CH2, CH2N, CH3, CH3N] = DutyCaculation(CNT, Tcomp1, Tcomp2, Tcomp3)

% CH1
if CNT < Tcomp1
    CH1 = 0;
    CH1N = 1;
else
    CH1 = 1;
    CH1N = 0;
end

% CH2
if CNT < Tcomp2
    CH2 = 0;
    CH2N = 1;
else
    CH2 = 1;
    CH2N = 0;
end

% CH3
if CNT < Tcomp3
    CH3 = 0;
    CH3N = 1;
else
    CH3 = 1;
    CH3N = 0;
end

== matlab function FOC/SVPWM/PWM SectorJudge ==
  data: A input; N output; B input; C input
function N = SectorJudge(A, B, C)


N = 0;
% if (A > 0)
%     A = 1
% end
% if (A < 0 )
%     A = 0
% end
% if (B > 0)
%     B = 1
% end
% if (B < 0 )
%     B = 0
% end
% if (C > 0)
%     C = 1
% end
% if (C < 0 )
%     C = 0
% end
% N = A + 2*B + 4*C

if (A>0)
    N = N + 1
end
if (B > 0)
    N = N + 2
end
if (C > 0)
    N = N + 4
end

== matlab function FOC/SVPWM/PWM CCRCaculation ==
  data: N input; Tcomp1 output; Ta input; Tb input; Tpwm input; Tcomp2 output; Tcomp3 output
function [Tcomp1, Tcomp2, Tcomp3] = CCRCaculation(N, Ta, Tb, Tpwm)

Tcomp1 = double(0);
Tcomp2 = double(0);
Tcomp3 = double(0);

Ttemp = Ta + Tb;
if (Ttemp > Tpwm)
    Ta = Ta / Ttemp * Tpwm;
    Tb = Tb / Ttemp * Tpwm;
end
value1 = (Tpwm - Ta - Tb) / 4.0;
value2 = value1 + Ta / 2.0;
value3 = value2 + Tb / 2.0;

switch(N)
    case 3
        Tcomp1 = value1;
        Tcomp2 = value2;
        Tcomp3 = value3;
    case 1
        Tcomp1 = value2;
        Tcomp2 = value1;
        Tcomp3 = value3;

    case 5
        Tcomp1 = value3;
        Tcomp2 = value1;
        Tcomp3 = value2;
    case 4
        Tcomp1 = value3;
        Tcomp2 = value2;
        Tcomp3 = value1;
    case 6
        Tcomp1 = value2;
        Tcomp2 = value3;
        Tcomp3 = value1;
    case 2
        Tcomp1 = value1;
        Tcomp2 = value3;
        Tcomp3 = value2;
end

== matlab function FOC/SVPWM/PWM VectorCaculation ==
  data: N input; Ta output; Valpa input; Vbeta input; Udc input; Tpwm input; Tb output
function [Ta, Tb] = SectorCaculation(N, Valpa, Vbeta, Udc, Tpwm)

Ta = double(0);
Tb = double(0);

X = (sqrt(3) * Tpwm) / Udc * Vbeta; % 扇区控制时间 系数1
Y = (sqrt(3) * Tpwm) / Udc * ((sqrt(3) / 2) * Valpa - (1/2) * Vbeta);%  系数2
Z = (sqrt(3) * Tpwm) / Udc * (-(sqrt(3) / 2) * Valpa - (1/2) * Vbeta);%  系数3

if (N == 3)
    Ta = Y;
    Tb = X;
end
if (N == 1) % 偶数扇区 Ta和Tb要交换位置
    Ta = -Y;
    Tb = -Z;
end
if (N == 5)
    Ta = X;
    Tb = Z;
end
if (N == 4)
    Ta = -X;
    Tb = -Y;
end
if (N == 6)
    Ta = Z;
    Tb = Y;
end
if (N == 2)
    Ta = -Z;
    Tb = -X;
end
